simulink model "MdXX_StatusToNetWork"  (R2024b)
settings: Solver=FixedStepDiscrete  StartTime=0.0  StopTime=10.0  FixedStep=0.01  RelTol=1e-3
undefined symbols (not defined in the file or in its folder): KeSMSbSRSPosNumConfig_Val
(part 2 of 2)

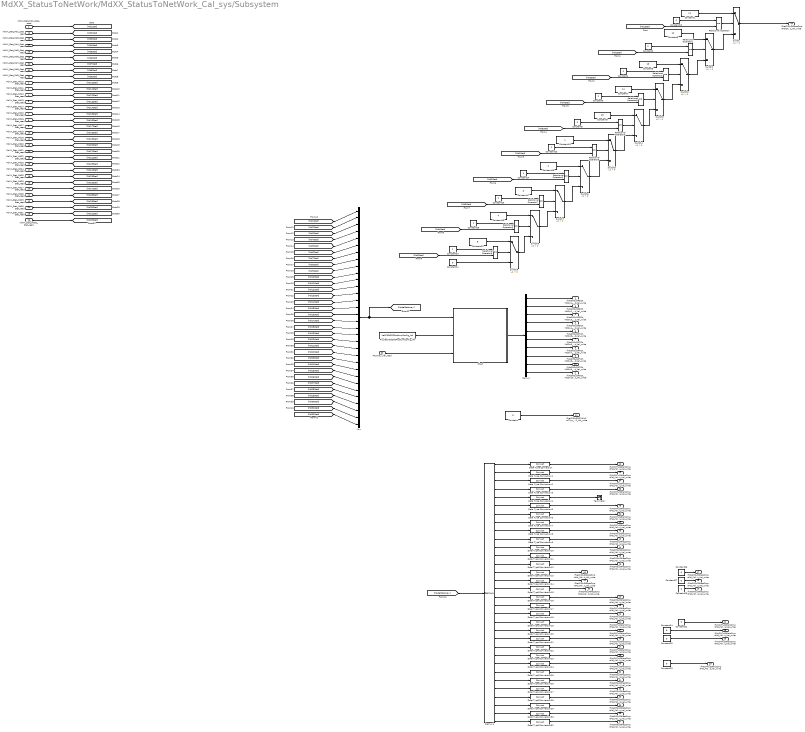
== system MdXX_StatusToNetWork/MdXX_StatusToNetWork_Cal_sys/Subsystem ==
  MdXX_Stat_Md1_Stat_read : Inport
  MdXX_Stat_Md10_Stat_read : Inport  Port=2
  MdXX_Stat_Md11_Stat_read : Inport  Port=3
  MdXX_Stat_Md12_Stat_read : Inport  Port=4
  MdXX_Stat_Md13_Stat_read : Inport  Port=5
  MdXX_Stat_Md14_Stat_read : Inport  Port=6
  MdXX_Stat_Md15_Stat_read : Inport  Port=7
  MdXX_Stat_Md16_Stat_read : Inport  Port=8
  MdXX_Stat_Md17_Stat_read : Inport  Port=9
  MdXX_Stat_Md18_Stat_read : Inport  Port=10
  MdXX_Stat_Md19_Stat_read : Inport  Port=11
  MdXX_Stat_Md2_Stat_read : Inport  Port=12
  MdXX_Stat_Md20_Stat_read : Inport  Port=13
  MdXX_Stat_Md21_Stat_read : Inport  Port=14
  MdXX_Stat_Md22_Stat_read : Inport  Port=15
  MdXX_Stat_Md23_Stat_read : Inport  Port=16
  MdXX_Stat_Md24_Stat_read : Inport  Port=17
  MdXX_Stat_Md25_Stat_read : Inport  Port=18
  MdXX_Stat_Md26_Stat_read : Inport  Port=19
  MdXX_Stat_Md27_Stat_read : Inport  Port=20
  MdXX_Stat_Md28_Stat_read : Inport  Port=21
  MdXX_Stat_Md29_Stat_read : Inport  Port=22
  MdXX_Stat_Md3_Stat_read : Inport  Port=23
  MdXX_Stat_Md30_Stat_read : Inport  Port=24
  MdXX_Stat_Md31_Stat_read : Inport  Port=25
  MdXX_Stat_Md32_Stat_read : Inport  Port=26
  MdXX_Stat_Md4_Stat_read : Inport  Port=27
  MdXX_Stat_Md5_Stat_read : Inport  Port=28
  MdXX_Stat_Md6_Stat_read : Inport  Port=29
  MdXX_Stat_Md7_Stat_read : Inport  Port=30
  MdXX_Stat_Md8_Stat_read : Inport  Port=31
  MdXX_Stat_Md9_Stat_read : Inport  Port=32
  PosArray_Val_read : Inport  Port=33
  Chart : Stateflow chart  TreatAsAtomicUnit=on
  Constant : Constant  Value=3  OutDataTypeStr=uint8
  Constant1 : Constant  Value=11  OutDataTypeStr=uint8
  Constant{2,4,6,8,10,15} (6 alike) : Constant  Value=2  OutDataTypeStr=uint8
  Constant{11,22..28} (8 alike) : Constant  Value=0  OutDataTypeStr=uint8
  Constant{12..14,16,18,20} (6 alike) : Constant  OutDataTypeStr=uint8
  Constant17 : Constant  Value=3  OutDataTypeStr=uint8
  Constant19 : Constant  Value=4  OutDataTypeStr=uint8
  Constant21 : Constant  Value=5  OutDataTypeStr=uint8
  Constant3 : Constant  Value=12  OutDataTypeStr=uint8
  Constant5 : Constant  Value=13  OutDataTypeStr=uint8
  Constant7 : Constant  Value=14  OutDataTypeStr=uint8
  Constant9 : Constant  Value=15  OutDataTypeStr=uint8
  Data Type Conversion{,1..31} (32 alike) : DataTypeConversion  SaturateOnIntegerOverflow=off  RndMeth=Floor
  Demux : Demux  Outputs=10
  Demux1 : Demux  Outputs=32
  Mux : Mux  Inputs=32
  PA_KeSMSbSRSPosNumConfig_Val : Constant  Value=KeSMSbSRSPosNumConfig_Val
  Relational Operator{,1..9} (10 alike) : RelationalOperator  Operator===  OutDataTypeStr=boolean  RndMeth=Simplest  InputSameDT=off
  Switch{,1..9} (10 alike) : Switch  Criteria=u2 > Threshold  SaturateOnIntegerOverflow=off  InputSameDT=off
  Terminator : Terminator
  IfVeSMSuSRSCrt_MdSw1_Stat_Val_write : Outport  VectorParamsAs1DForOutWhenUnconnected=off
      settings: EnsureOutportIsVirtual=on
  IfVeSMSuSRSCrt_MdSw10_Stat_Val_write : Outport  Port=2  VectorParamsAs1DForOutWhenUnconnected=off
      settings: EnsureOutportIsVirtual=on
  IfVeSMSuSRSCrt_MdSw2_Stat_Val_write : Outport  Port=3  VectorParamsAs1DForOutWhenUnconnected=off
      settings: EnsureOutportIsVirtual=on
  IfVeSMSuSRSCrt_MdSw3_Stat_Val_write : Outport  Port=4  VectorParamsAs1DForOutWhenUnconnected=off
      settings: EnsureOutportIsVirtual=on
  IfVeSMSuSRSCrt_MdSw4_Stat_Val_write : Outport  Port=5  VectorParamsAs1DForOutWhenUnconnected=off
      settings: EnsureOutportIsVirtual=on
  IfVeSMSuSRSCrt_MdSw5_Stat_Val_write : Outport  Port=6  VectorParamsAs1DForOutWhenUnconnected=off
      settings: EnsureOutportIsVirtual=on
  IfVeSMSuSRSCrt_MdSw6_Stat_Val_write : Outport  Port=7  VectorParamsAs1DForOutWhenUnconnected=off
      settings: EnsureOutportIsVirtual=on
  IfVeSMSuSRSCrt_MdSw7_Stat_Val_write : Outport  Port=8  VectorParamsAs1DForOutWhenUnconnected=off
      settings: EnsureOutportIsVirtual=on
  IfVeSMSuSRSCrt_MdSw8_Stat_Val_write : Outport  Port=9  VectorParamsAs1DForOutWhenUnconnected=off
      settings: EnsureOutportIsVirtual=on
  IfVeSMSuSRSCrt_MdSw9_Stat_Val_write : Outport  Port=10  VectorParamsAs1DForOutWhenUnconnected=off
      settings: EnsureOutportIsVirtual=on
  IfVeSMSuSRSCrtMdIndTyp_67_2_Val_write : Outport  Port=11  VectorParamsAs1DForOutWhenUnconnected=off
      settings: EnsureOutportIsVirtual=on
  IfVeSMSuStPassCmprtMd_Md1_CrtStat_Val_write : Outport  Port=12  VectorParamsAs1DForOutWhenUnconnected=off
      settings: EnsureOutportIsVirtual=on
  IfVeSMSuStPassCmprtMd_Md10_CrtStat_Val_write : Outport  Port=13  VectorParamsAs1DForOutWhenUnconnected=off
      settings: EnsureOutportIsVirtual=on
  IfVeSMSuStPassCmprtMd_Md11_CrtStat_Val_write : Outport  Port=14  VectorParamsAs1DForOutWhenUnconnected=off
      settings: EnsureOutportIsVirtual=on
  IfVeSMSuStPassCmprtMd_Md12_CrtStat_Val_write : Outport  Port=15  VectorParamsAs1DForOutWhenUnconnected=off
      settings: EnsureOutportIsVirtual=on
  IfVeSMSuStPassCmprtMd_Md13_CrtStat_Val_write : Outport  Port=16  VectorParamsAs1DForOutWhenUnconnected=off
      settings: EnsureOutportIsVirtual=on
  IfVeSMSuStPassCmprtMd_Md14_CrtStat_Val_write : Outport  Port=17  VectorParamsAs1DForOutWhenUnconnected=off
      settings: EnsureOutportIsVirtual=on
  IfVeSMSuStPassCmprtMd_Md15_CrtStat_Val_write : Outport  Port=18  VectorParamsAs1DForOutWhenUnconnected=off
      settings: EnsureOutportIsVirtual=on
  IfVeSMSuStPassCmprtMd_Md16_CrtStat_Val_write : Outport  Port=19  VectorParamsAs1DForOutWhenUnconnected=off
      settings: EnsureOutportIsVirtual=on
  IfVeSMSuStPassCmprtMd_Md17_CrtStat_Val_write : Outport  Port=20  VectorParamsAs1DForOutWhenUnconnected=off
      settings: EnsureOutportIsVirtual=on
  IfVeSMSuStPassCmprtMd_Md18_CrtStat_Val_write : Outport  Port=21  VectorParamsAs1DForOutWhenUnconnected=off
      settings: EnsureOutportIsVirtual=on
  IfVeSMSuStPassCmprtMd_Md19_CrtStat_Val_write : Outport  Port=22  VectorParamsAs1DForOutWhenUnconnected=off
      settings: EnsureOutportIsVirtual=on
  IfVeSMSuStPassCmprtMd_Md2_CrtStat_Val_write : Outport  Port=23  VectorParamsAs1DForOutWhenUnconnected=off
      settings: EnsureOutportIsVirtual=on
  IfVeSMSuStPassCmprtMd_Md20_CrtStat_Val_write : Outport  Port=24  VectorParamsAs1DForOutWhenUnconnected=off
      settings: EnsureOutportIsVirtual=on
  IfVeSMSuStPassCmprtMd_Md21_CrtStat_Val_write : Outport  Port=25  VectorParamsAs1DForOutWhenUnconnected=off
      settings: EnsureOutportIsVirtual=on
  IfVeSMSuStPassCmprtMd_Md22_CrtStat_Val_write : Outport  Port=26  VectorParamsAs1DForOutWhenUnconnected=off
      settings: EnsureOutportIsVirtual=on
  IfVeSMSuStPassCmprtMd_Md23_CrtStat_Val_write : Outport  Port=27  VectorParamsAs1DForOutWhenUnconnected=off
      settings: EnsureOutportIsVirtual=on
  IfVeSMSuStPassCmprtMd_Md24_CrtStat_Val_write : Outport  Port=28  VectorParamsAs1DForOutWhenUnconnected=off
      settings: EnsureOutportIsVirtual=on
  IfVeSMSuStPassCmprtMd_Md25_CrtStat_Val_write : Outport  Port=29  VectorParamsAs1DForOutWhenUnconnected=off
      settings: EnsureOutportIsVirtual=on
  IfVeSMSuStPassCmprtMd_Md26_CrtStat_Val_write : Outport  Port=30  VectorParamsAs1DForOutWhenUnconnected=off
      settings: EnsureOutportIsVirtual=on
  IfVeSMSuStPassCmprtMd_Md27_CrtStat_Val_write : Outport  Port=31  VectorParamsAs1DForOutWhenUnconnected=off
      settings: EnsureOutportIsVirtual=on
  IfVeSMSuStPassCmprtMd_Md28_CrtStat_Val_write : Outport  Port=32  VectorParamsAs1DForOutWhenUnconnected=off
      settings: EnsureOutportIsVirtual=on
  IfVeSMSuStPassCmprtMd_Md29_CrtStat_Val_write : Outport  Port=33  VectorParamsAs1DForOutWhenUnconnected=off
      settings: EnsureOutportIsVirtual=on
  IfVeSMSuStPassCmprtMd_Md3_CrtStat_Val_write : Outport  Port=34  VectorParamsAs1DForOutWhenUnconnected=off
      settings: EnsureOutportIsVirtual=on
  IfVeSMSuStPassCmprtMd_Md30_CrtStat_Val_write : Outport  Port=35  VectorParamsAs1DForOutWhenUnconnected=off
      settings: EnsureOutportIsVirtual=on
  IfVeSMSuStPassCmprtMd_Md31_CrtStat_Val_write : Outport  Port=36  VectorParamsAs1DForOutWhenUnconnected=off
      settings: EnsureOutportIsVirtual=on
  IfVeSMSuStPassCmprtMd_Md32_CrtStat_Val_write : Outport  Port=37  VectorParamsAs1DForOutWhenUnconnected=off
      settings: EnsureOutportIsVirtual=on
  IfVeSMSuStPassCmprtMd_Md4_CrtStat_Val_write : Outport  Port=38  VectorParamsAs1DForOutWhenUnconnected=off
      settings: EnsureOutportIsVirtual=on
  IfVeSMSuStPassCmprtMd_Md5_CrtStat_Val_write : Outport  Port=39  VectorParamsAs1DForOutWhenUnconnected=off
      settings: EnsureOutportIsVirtual=on
  IfVeSMSuStPassCmprtMd_Md6_CrtStat_Val_write : Outport  Port=40  VectorParamsAs1DForOutWhenUnconnected=off
      settings: EnsureOutportIsVirtual=on
  IfVeSMSuStPassCmprtMd_Md7_CrtStat_Val_write : Outport  Port=41  VectorParamsAs1DForOutWhenUnconnected=off
      settings: EnsureOutportIsVirtual=on
  IfVeSMSuStPassCmprtMd_Md8_CrtStat_Val_write : Outport  Port=42  VectorParamsAs1DForOutWhenUnconnected=off
      settings: EnsureOutportIsVirtual=on
  IfVeSMSuStPassCmprtMd_Md9_CrtStat_Val_write : Outport  Port=43  VectorParamsAs1DForOutWhenUnconnected=off
      settings: EnsureOutportIsVirtual=on
  IfVeSMSuStPassCmprtMdCrtMdStat_Val_write : Outport  Port=44  VectorParamsAs1DForOutWhenUnconnected=off
      settings: EnsureOutportIsVirtual=on
  IfVeSMSuStPassCmprtMd_Md53_CrtStat_Val_write : Outport  Port=45  VectorParamsAs1DForOutWhenUnconnected=off
      settings: EnsureOutportIsVirtual=on
  IfVeSMSuStPassCmprtMd_Md56_CrtStat_Val_write : Outport  Port=46  VectorParamsAs1DForOutWhenUnconnected=off
      settings: EnsureOutportIsVirtual=on
  IfVeSMSuStPassCmprtMd_Md57_CrtStat_Val_write : Outport  Port=47  VectorParamsAs1DForOutWhenUnconnected=off
      settings: EnsureOutportIsVirtual=on
  IfVeSMSuStPassCmprtMd_Md58_CrtStat_Val_write : Outport  Port=48  VectorParamsAs1DForOutWhenUnconnected=off
      settings: EnsureOutportIsVirtual=on
  IfVeSMSuStPassCmprtMd_Md61_CrtStat_Val_write : Outport  Port=49  VectorParamsAs1DForOutWhenUnconnected=off
      settings: EnsureOutportIsVirtual=on
  IfVeSMSuStPassCmprtMd_Md62_CrtStat_Val_write : Outport  Port=50  VectorParamsAs1DForOutWhenUnconnected=off
      settings: EnsureOutportIsVirtual=on
  wires:
  Constant/1 -> IfVeSMSuSRSCrtMdIndTyp_67_2_Val_write/1
  Switch/1 -> IfVeSMSuStPassCmprtMdCrtMdStat_Val_write/1
  MdXX_Stat_Md19_Stat_read/1 -> [Md19Stat]
  MdXX_Stat_Md31_Stat_read/1 -> [Md31Stat]
  MdXX_Stat_Md14_Stat_read/1 -> [Md14Stat]
  MdXX_Stat_Md15_Stat_read/1 -> [Md15Stat]
  MdXX_Stat_Md23_Stat_read/1 -> [Md23Stat]
  MdXX_Stat_Md30_Stat_read/1 -> [Md30Stat]
  MdXX_Stat_Md28_Stat_read/1 -> [Md28Stat]
  MdXX_Stat_Md26_Stat_read/1 -> [Md26Stat]
  MdXX_Stat_Md27_Stat_read/1 -> [Md27Stat]
  MdXX_Stat_Md21_Stat_read/1 -> [Md21Stat]
  MdXX_Stat_Md25_Stat_read/1 -> [Md25Stat]
  MdXX_Stat_Md22_Stat_read/1 -> [Md22Stat]
  MdXX_Stat_Md2_Stat_read/1 -> [Md2Stat]
  MdXX_Stat_Md13_Stat_read/1 -> [Md13Stat]
  MdXX_Stat_Md17_Stat_read/1 -> [Md17Stat]
  MdXX_Stat_Md16_Stat_read/1 -> [Md16Stat]
  MdXX_Stat_Md29_Stat_read/1 -> [Md29Stat]
  MdXX_Stat_Md18_Stat_read/1 -> [Md18Stat]
  MdXX_Stat_Md8_Stat_read/1 -> [Md8Stat]
  MdXX_Stat_Md5_Stat_read/1 -> [Md5Stat]
  MdXX_Stat_Md3_Stat_read/1 -> [Md3Stat]
  MdXX_Stat_Md11_Stat_read/1 -> [Md11Stat]
  MdXX_Stat_Md12_Stat_read/1 -> [Md12Stat]
  MdXX_Stat_Md20_Stat_read/1 -> [Md20Stat]
  MdXX_Stat_Md4_Stat_read/1 -> [Md4Stat]
  MdXX_Stat_Md32_Stat_read/1 -> [Md32Stat]
  MdXX_Stat_Md9_Stat_read/1 -> [Md9Stat]
  MdXX_Stat_Md6_Stat_read/1 -> [Md6Stat]
  MdXX_Stat_Md10_Stat_read/1 -> [Md10Stat]
  MdXX_Stat_Md7_Stat_read/1 -> [Md7Stat]
  MdXX_Stat_Md1_Stat_read/1 -> [Md1Stat]
  MdXX_Stat_Md24_Stat_read/1 -> [Md24Stat]
  Constant11/1 -> Switch9/3
  Switch6/1 -> Switch5/3
  Constant16/1 -> Relational Operator7/1
  Switch1/1 -> Switch/3
  Constant19/1 -> Switch8/1
  Switch5/1 -> Switch4/3
  [Md2Stat] -> Relational Operator1/2
  [Md4Stat] -> Relational Operator3/2
  Relational Operator8/1 -> Switch8/2
  Switch9/1 -> Switch8/3
  Constant5/1 -> Switch2/1
  Switch4/1 -> Switch3/3
  [Md3Stat] -> Relational Operator7/2
  Constant2/1 -> Relational Operator1/1
  Constant13/1 -> Relational Operator5/1
  Constant21/1 -> Switch9/1
  Constant9/1 -> Switch4/1
  Switch3/1 -> Switch2/3
  [Md1Stat] -> Relational Operator/2
  Constant4/1 -> Relational Operator2/1
  Constant6/1 -> Relational Operator3/1
  [Md5Stat] -> Relational Operator4/2
  Relational Operator1/1 -> Switch1/2
  Constant7/1 -> Switch3/1
  Relational Operator7/1 -> Switch7/2
  Constant10/1 -> Relational Operator/1
  Constant17/1 -> Switch7/1
  Switch2/1 -> Switch1/3
  Constant15/1 -> Switch6/1
  Switch8/1 -> Switch7/3
  Relational Operator/1 -> Switch/2
  Relational Operator3/1 -> Switch3/2
  Constant20/1 -> Relational Operator9/1
  Constant18/1 -> Relational Operator8/1
  [Md5Stat] -> Relational Operator9/2
  Relational Operator9/1 -> Switch9/2
  Constant12/1 -> Switch5/1
  Switch7/1 -> Switch6/3
  Constant3/1 -> Switch1/1
  [Md1Stat] -> Relational Operator5/2
  [Md3Stat] -> Relational Operator2/2
  Relational Operator2/1 -> Switch2/2
  Relational Operator5/1 -> Switch5/2
  [Md2Stat] -> Relational Operator6/2
  Constant14/1 -> Relational Operator6/1
  Constant1/1 -> Switch/1
  Constant8/1 -> Relational Operator4/1
  [Md4Stat] -> Relational Operator8/2
  Relational Operator6/1 -> Switch6/2
  Relational Operator4/1 -> Switch4/2
  Demux/6 -> IfVeSMSuSRSCrt_MdSw6_Stat_Val_write/1
  Demux/5 -> IfVeSMSuSRSCrt_MdSw5_Stat_Val_write/1
  Demux/4 -> IfVeSMSuSRSCrt_MdSw4_Stat_Val_write/1
  Chart/1(ModeStatSRSswArray) -> Demux/1
  Demux/1 -> IfVeSMSuSRSCrt_MdSw1_Stat_Val_write/1
  Demux/2 -> IfVeSMSuSRSCrt_MdSw2_Stat_Val_write/1
  Demux/9 -> IfVeSMSuSRSCrt_MdSw9_Stat_Val_write/1
  Demux/8 -> IfVeSMSuSRSCrt_MdSw8_Stat_Val_write/1
  PA_KeSMSbSRSPosNumConfig_Val/1 -> Chart/2(KeSMSbSRSPosNumConfig)
  Mux/1 -> [ModeStatArray], Chart/1(ModeStatArray)
  Demux/10 -> IfVeSMSuSRSCrt_MdSw10_Stat_Val_write/1
  PosArray_Val_read/1 -> Chart/3(PosArray)
  Demux/7 -> IfVeSMSuSRSCrt_MdSw7_Stat_Val_write/1
  Demux/3 -> IfVeSMSuSRSCrt_MdSw3_Stat_Val_write/1
  [Md1Stat] -> Mux/1
  [Md2Stat] -> Mux/2
  [Md3Stat] -> Mux/3
  [Md4Stat] -> Mux/4
  [Md5Stat] -> Mux/5
  [Md6Stat] -> Mux/6
  [Md7Stat] -> Mux/7
  [Md8Stat] -> Mux/8
  [Md9Stat] -> Mux/9
  [Md10Stat] -> Mux/10
  [Md11Stat] -> Mux/11
  [Md12Stat] -> Mux/12
  [Md13Stat] -> Mux/13
  [Md14Stat] -> Mux/14
  [Md15Stat] -> Mux/15
  [Md16Stat] -> Mux/16
  [Md17Stat] -> Mux/17
  [Md18Stat] -> Mux/18
  [Md19Stat] -> Mux/19
  [Md20Stat] -> Mux/20
  [Md21Stat] -> Mux/21
  [Md22Stat] -> Mux/22
  [Md23Stat] -> Mux/23
  [Md24Stat] -> Mux/24
  [Md25Stat] -> Mux/25
  [Md26Stat] -> Mux/26
  [Md27Stat] -> Mux/27
  [Md28Stat] -> Mux/28
  [Md29Stat] -> Mux/29
  [Md30Stat] -> Mux/30
  [Md31Stat] -> Mux/31
  [Md32Stat] -> Mux/32
  Demux1/15 -> Data Type Conversion14/1
  Demux1/16 -> Data Type Conversion15/1
  Demux1/14 -> Data Type Conversion13/1
  Demux1/17 -> Data Type Conversion16/1
  Demux1/18 -> Data Type Conversion17/1
  Demux1/21 -> Data Type Conversion20/1
  Demux1/22 -> Data Type Conversion21/1
  Demux1/12 -> Data Type Conversion11/1
  Demux1/13 -> Data Type Conversion12/1
  Demux1/19 -> Data Type Conversion18/1
  Demux1/20 -> Data Type Conversion19/1
  Demux1/23 -> Data Type Conversion22/1
  Demux1/10 -> Data Type Conversion9/1
  Demux1/11 -> Data Type Conversion10/1
  Demux1/24 -> Data Type Conversion23/1
  Demux1/25 -> Data Type Conversion24/1
  Demux1/9 -> Data Type Conversion8/1
  Demux1/26 -> Data Type Conversion25/1
  Demux1/27 -> Data Type Conversion26/1
  Demux1/8 -> Data Type Conversion7/1
  Demux1/28 -> Data Type Conversion27/1
  Demux1/6 -> Data Type Conversion5/1
  Demux1/7 -> Data Type Conversion6/1
  Demux1/29 -> Data Type Conversion28/1
  Demux1/30 -> Data Type Conversion29/1
  Demux1/31 -> Data Type Conversion30/1
  Demux1/1 -> Data Type Conversion/1
  Demux1/2 -> Data Type Conversion1/1
  Demux1/3 -> Data Type Conversion2/1
  Demux1/4 -> Data Type Conversion3/1
  Demux1/5 -> Data Type Conversion4/1
  Demux1/32 -> Data Type Conversion31/1
  [ModeStatArray] -> Demux1/1
  Data Type Conversion/1 -> IfVeSMSuStPassCmprtMd_Md1_CrtStat_Val_write/1
  Data Type Conversion1/1 -> IfVeSMSuStPassCmprtMd_Md2_CrtStat_Val_write/1
  Data Type Conversion2/1 -> IfVeSMSuStPassCmprtMd_Md3_CrtStat_Val_write/1
  Data Type Conversion3/1 -> IfVeSMSuStPassCmprtMd_Md4_CrtStat_Val_write/1
  Data Type Conversion7/1 -> IfVeSMSuStPassCmprtMd_Md8_CrtStat_Val_write/1
  Data Type Conversion8/1 -> IfVeSMSuStPassCmprtMd_Md9_CrtStat_Val_write/1
  Data Type Conversion9/1 -> IfVeSMSuStPassCmprtMd_Md10_CrtStat_Val_write/1
  Data Type Conversion10/1 -> IfVeSMSuStPassCmprtMd_Md11_CrtStat_Val_write/1
  Data Type Conversion11/1 -> IfVeSMSuStPassCmprtMd_Md12_CrtStat_Val_write/1
  Data Type Conversion12/1 -> IfVeSMSuStPassCmprtMd_Md13_CrtStat_Val_write/1
  Data Type Conversion16/1 -> IfVeSMSuStPassCmprtMd_Md17_CrtStat_Val_write/1
  Data Type Conversion18/1 -> IfVeSMSuStPassCmprtMd_Md19_CrtStat_Val_write/1
  Data Type Conversion19/1 -> IfVeSMSuStPassCmprtMd_Md20_CrtStat_Val_write/1
  Data Type Conversion22/1 -> IfVeSMSuStPassCmprtMd_Md23_CrtStat_Val_write/1
  Data Type Conversion23/1 -> IfVeSMSuStPassCmprtMd_Md24_CrtStat_Val_write/1
  Data Type Conversion25/1 -> IfVeSMSuStPassCmprtMd_Md26_CrtStat_Val_write/1
  Data Type Conversion26/1 -> IfVeSMSuStPassCmprtMd_Md27_CrtStat_Val_write/1
  Data Type Conversion27/1 -> IfVeSMSuStPassCmprtMd_Md28_CrtStat_Val_write/1
  Data Type Conversion28/1 -> IfVeSMSuStPassCmprtMd_Md29_CrtStat_Val_write/1
  Data Type Conversion29/1 -> IfVeSMSuStPassCmprtMd_Md30_CrtStat_Val_write/1
  Data Type Conversion30/1 -> IfVeSMSuStPassCmprtMd_Md31_CrtStat_Val_write/1
  Data Type Conversion31/1 -> IfVeSMSuStPassCmprtMd_Md32_CrtStat_Val_write/1
  Data Type Conversion17/1 -> IfVeSMSuStPassCmprtMd_Md53_CrtStat_Val_write/1
  Data Type Conversion24/1 -> IfVeSMSuStPassCmprtMd_Md56_CrtStat_Val_write/1
  Constant22/1 -> IfVeSMSuStPassCmprtMd_Md18_CrtStat_Val_write/1
  Constant23/1 -> IfVeSMSuStPassCmprtMd_Md25_CrtStat_Val_write/1
  Data Type Conversion21/1 -> IfVeSMSuStPassCmprtMd_Md58_CrtStat_Val_write/1
  Data Type Conversion20/1 -> IfVeSMSuStPassCmprtMd_Md57_CrtStat_Val_write/1
  Constant24/1 -> IfVeSMSuStPassCmprtMd_Md21_CrtStat_Val_write/1
  Constant25/1 -> IfVeSMSuStPassCmprtMd_Md22_CrtStat_Val_write/1
  Data Type Conversion5/1 -> IfVeSMSuStPassCmprtMd_Md61_CrtStat_Val_write/1
  Data Type Conversion6/1 -> IfVeSMSuStPassCmprtMd_Md62_CrtStat_Val_write/1
  Data Type Conversion4/1 -> Terminator/1
  Constant26/1 -> IfVeSMSuStPassCmprtMd_Md14_CrtStat_Val_write/1
  Constant27/1 -> IfVeSMSuStPassCmprtMd_Md15_CrtStat_Val_write/1
  Constant28/1 -> IfVeSMSuStPassCmprtMd_Md16_CrtStat_Val_write/1
  Data Type Conversion13/1 -> IfVeSMSuStPassCmprtMd_Md6_CrtStat_Val_write/1
  Data Type Conversion14/1 -> IfVeSMSuStPassCmprtMd_Md7_CrtStat_Val_write/1
  Data Type Conversion15/1 -> IfVeSMSuStPassCmprtMd_Md5_CrtStat_Val_write/1

== stateflow chart MdXX_StatusToNetWork/MdXX_StatusToNetWork_Cal_sys/Subsystem/Chart ==
  (default) -> (junction 5) : {i=0;}
  (junction 7) -> (junction 22) [order 1] : [PosArray[i+1]<1]
  (junction 5) -> (junction 7) [order 1] : [i<KeSMSbSRSPosNumConfig]
  (junction 7) -> (junction 9) [order 2] : {
      | ModeStatSRSswArray[i]=ModeStatArray[PosArray[i+1]-1];
      | }
  (junction 22) -> (junction 24) : {
      | ModeStatSRSswArray[i]=0;
      | }
  (junction 9) -> (junction 5) : {i=i+1;}
  (junction 5) -> (junction 12) [order 2]
  (junction 24) -> (junction 9)
  (junction 12) -> (junction 14) [order 1] : [i<10]
  (junction 14) -> (junction 16) : {
      | ModeStatSRSswArray[i]=0;
      | }
  (junction 16) -> (junction 12) : {i=i+1;}
  (junction 12) -> (junction 19) [order 2]
  data: ModeStatArray input uint8 size=32; KeSMSbSRSPosNumConfig input uint8; i local uint8; ModeStatSRSswArray output uint8 size=10; PosArray input uint8 size=11
